simulink model "geo_projective"  (Simulink 8.3)
settings: Solver=FixedStepDiscrete  StartTime=0.0  StopTime=inf  RelTol=1e-3
undefined symbols (not defined in the file): gray
libraries: visionsinks x2, visiongeotforms x1, visionsources x1
settings Model: Creator=FxMain  LastModifiedBy=Vasilis
settings OptimizationCC: ExpressionDepthLimit=2147483647
settings DebuggingCC: FcnCallInpInsideContextMsg=UseLocalSettings

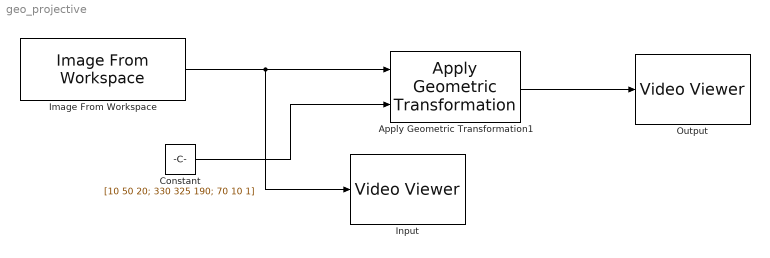
== system geo_projective ==
  Apply Geometric Transformation1 : visiongeotforms/Apply Geometric Transformation  tformSource=Input port  tformValue=[1 0 0; 0 1 0; 0 0 1]  approxProjectiveFlag=off  errorTolerance=1.0  roiMethod=Whole input image  roiSource=Specify via dialog  roiBBox=[1 1 256 128]  roiVertice=[1 1 12 10 22 20]  inputClipFlag=off  interpolationMethod=Bilinear  fillValue=0  viewPortMethod=Same as input image  outputSize=[5120 5120]  outputLoc=[1 1]  outputClipFlag=off
  Constant : Constant  Value=[10 50 20; 330 325 190; 70 10 1]
      settings: SamplingMode=Frame based
  Image From Workspace : visionsources/Image From Workspace  Tag=vipblks_nd  ImageValue=img  Ts=inf  imagePorts=One multidimensional signal  ImageDataType=Inherit from 'Value'  Signed=on  WordLength=16  sdImageDataType=sfix(16)  FractionLengthMode=User-defined  FractionLength=15  OutPortLabels=R|G|B
  Input : visionsinks/Video Viewer  inputType=Obsolete7b  imagePorts=One multidimensional signal  useColorMap=off  colormapValue=gray(256)  specRange=on  minInputVal=0  maxInputVal=255  FigPos=[1 726 1366 626]  AxisZoom=on  trueSizedOnce=off  OpenAtMdlStart=on  DefaultConfigurationName=vipscopes.VideoViewerScopeCfg
  Output : visionsinks/Video Viewer  inputType=Obsolete7b  imagePorts=One multidimensional signal  useColorMap=off  colormapValue=gray(256)  specRange=on  minInputVal=0  maxInputVal=255  FigPos=[1677 979 959 866]  AxisZoom=on  trueSizedOnce=off  OpenAtMdlStart=on  DefaultConfigurationName=vipscopes.VideoViewerScopeCfg
  wires:
  Image From Workspace/1 -> Apply Geometric Transformation1/1, Input/1
  Constant/1 -> Apply Geometric Transformation1/2
  Apply Geometric Transformation1/1 -> Output/1
